simulink model "FDMA"  (R2018a)
settings: Solver=VariableStepAuto  StartTime=0.0  StopTime=10.0  RelTol=1e-3
libraries: dsparch4 x4
settings Model: Creator=DAWOOD  LastModifiedBy=DAWOOD

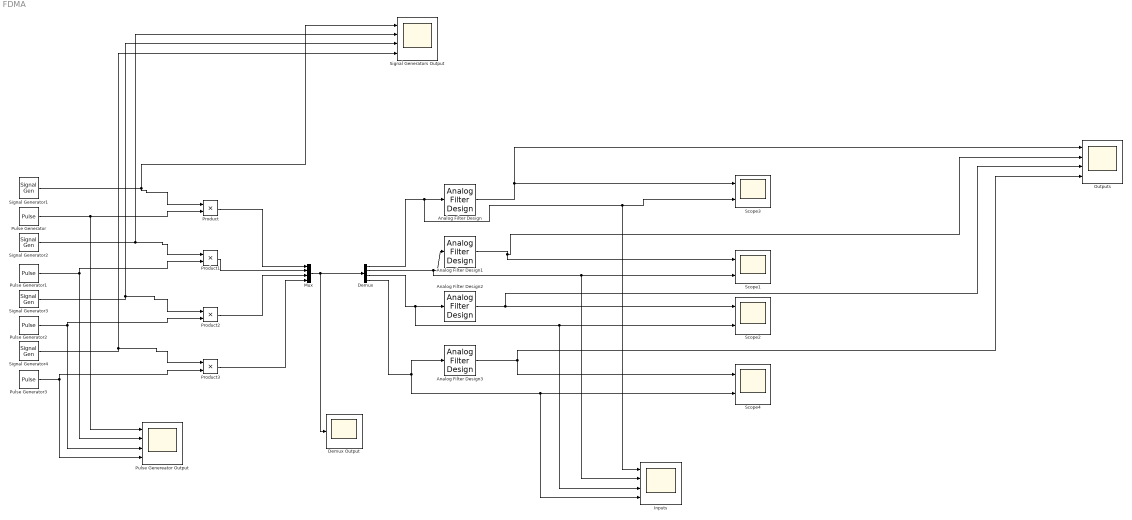
== system FDMA ==
  Analog Filter Design : dsparch4/Analog Filter Design  method=Butterworth  filttype=Lowpass  N=8  Wlo=2*pi  Whi=80  Rp=2  Rs=40
  Analog Filter Design1 : dsparch4/Analog Filter Design  method=Butterworth  filttype=Lowpass  N=8  Wlo=4*pi  Whi=80  Rp=2  Rs=40
  Analog Filter Design2 : dsparch4/Analog Filter Design  method=Butterworth  filttype=Lowpass  N=8  Wlo=6*pi  Whi=80  Rp=2  Rs=40
  Analog Filter Design3 : dsparch4/Analog Filter Design  method=Butterworth  filttype=Lowpass  N=8  Wlo=8*pi  Whi=80  Rp=2  Rs=40
  Demux : Demux
  Demux Output : Scope
  "Inputs " : Scope  NumInputPorts=4
  Mux : Mux
  "Outputs " : Scope  NumInputPorts=4
  Product{,1..3} (4 alike) : Product
  Pulse Generator{,1..3} (4 alike) : DiscretePulseGenerator  PulseType=Time based  Period=0.1  PulseWidth=5  PhaseDelay=0.1
  Pulse Genereator Output : Scope  NumInputPorts=4
  Scope{1..4} (4 alike) : Scope  NumInputPorts=2
  Signal Generator1 : SignalGenerator  Frequency=2*pi  Units=rad/sec
  Signal Generator2 : SignalGenerator  Frequency=4*pi  Units=rad/sec
  Signal Generator3 : SignalGenerator  Frequency=6*pi  Units=rad/sec
  Signal Generator4 : SignalGenerator  Frequency=8*pi  Units=rad/sec
  Signal Generators Output : Scope  NumInputPorts=4
  wires:
  Signal Generator1/1 -> Product/1, Signal Generators Output/1
  Pulse Generator/1 -> Product/2, Pulse Genereator Output/1
  Signal Generator2/1 -> Signal Generators Output/2, Product1/1
  Pulse Generator1/1 -> Product1/2, Pulse Genereator Output/2
  Signal Generator3/1 -> Product2/1, Signal Generators Output/3
  Pulse Generator2/1 -> Product2/2, Pulse Genereator Output/3
  Signal Generator4/1 -> Product3/1, Signal Generators Output/4
  Pulse Generator3/1 -> Product3/2, Pulse Genereator Output/4
  Product/1 -> Mux/1
  Product1/1 -> Mux/2
  Product2/1 -> Mux/3
  Product3/1 -> Mux/4
  Mux/1 -> Demux Output/1, Demux/1
  Demux/1 -> "Inputs "/1, Scope3/2, Analog Filter Design/1
  Demux/2 -> "Inputs "/2, Scope1/2, Analog Filter Design1/1
  Demux/3 -> "Inputs "/3, Scope2/2, Analog Filter Design2/1
  Demux/4 -> "Inputs "/4, Scope4/2, Analog Filter Design3/1
  Analog Filter Design1/1 -> "Outputs "/2, Scope1/1
  Analog Filter Design3/1 -> Scope4/1, "Outputs "/4
  Analog Filter Design/1 -> "Outputs "/1, Scope3/1
  Analog Filter Design2/1 -> "Outputs "/3, Scope2/1
